simulink model "testEmplanner_cs -copy"  (R2021b)
settings: Solver=ode5  StartTime=0.0  StopTime=30  FixedStep=1/1000  RelTol=1e-3
PreLoadFcn:
  | mbxruntime.callbacks.PreLoadFcn(bdroot);
PostLoadFcn:
  | mbxruntime.callbacks.PostLoadFcn(bdroot);
InitFcn:
  | mbxruntime.callbacks.InitFcn(bdroot);
StartFcn:
  | mbxruntime.callbacks.StartFcn(bdroot);
StopFcn:
  | mbxruntime.callbacks.StopFcn(bdroot);
model workspace (MAT data in the model file):
  mbox_table : object (value not decoded)
  model_closed = 0
  sim_status = 0
values from neighbouring files (symbols this model uses):
  c_factor = 43.75    [emplanner_init.m]
  cf = -175016    [emplanner_init.m]
  cr = -130634    [emplanner_init.m]
  global_path_x = [-1.1448 -0.145417744933 0.852705365581 1.84955224935 2.84511712279 3.83939835808 4.83239585569 5.82411007764 6.81454169183 7.80369144113 8.79156009523 9.77814843293 ... (3001 elements, 3001x1)]    [global_path.mat]
  global_path_y = [14.6488 14.6488 14.6488 14.6488 14.6488 14.6488 14.6488 14.6488 14.6488 14.6488 14.6488 14.6488 ... (3001 elements, 3001x1)]    [global_path.mat]
  KD_PID_distance = 0.0    (= 0)    [emplanner_init.m]
  KD_PID_speed = 0    [emplanner_init.m]
  KI_PID_distance = 0.0    (= 0)    [emplanner_init.m]
  KI_PID_speed = 0    [emplanner_init.m]
  KP_PID_distance = 0.5    [emplanner_init.m]
  KP_PID_speed = 1.8    [emplanner_init.m]
  la = 1.265    [emplanner_init.m]
  lb = 2.947-1.265    (= 1.682)    [emplanner_init.m]
  LQR_K1 = k(:,1)'    [emplanner_init.m]
  LQR_K2 = k(:,2)'    [emplanner_init.m]
  LQR_K3 = k(:,3)'    [emplanner_init.m]
  LQR_K4 = k(:,4)'    [emplanner_init.m]
  m = 2020    [emplanner_init.m]
  rack_displacement = [-39.14 , -37.2 , -35.29 , -33.43 , -31.6 , -29.81 , -28.06 , -26.34 , -24.66 ,      -23.01 , -21.38 , -19.79 , -18.23 , -16.69 , -15.18 , -13.7 , -12.23 , -10.8 , -9.38 , -7.98 ,     -6.61 , -5.25 , -3.91 , -2.59 , -1.29 , 0 , 1.27 , 2.54 , 3.78 , 5.02 , 6.24 , 7.46 , 8.66 ,      9.86 , 11.05 , 12.24 , 13.41 , 14.59 , 15.76 , 16.92 , 18.09 , 19.25 , 20.42 , 21.59 , 22.76 ,      23.93 , 25.11 , 26 ...(+26 chars)    [emplanner_init.m]
  right_wheel_ground = [-70 ,-67.2 , -64.4 , -61.6 , -58.8 , -56 , -53.2 , -50.4 , -47.6 , -44.8 , -42 ,      -39.2 , -36.4 , -33.6 , -30.8 , -28 , -25.2 , -22.4 , -19.6 , -16.8 , -14 , -11.2 , -8.4 , -5.6 ,      -2.8 , 0 , 2.8 , 5.6 , 8.4 , 11.2 , 14 , 16.8 , 19.6 , 22.4 , 25.2 , 28 , 30.8 , 33.6 , 36.4 ,      39.2 , 42 , 44.8 , 47.6 , 50.4 , 53.2 , 56 , 58.8 , 61.6 , 64.4 , 67.2 , 70 ]    [emplanner_init.m]
  vx_break_point = zeros(1,5000)    [emplanner_init.m]
undefined symbols (not defined in the file or in its folder): aubr, DiscIntNeverNeededParam, tablebr, vubr, warningInitialVelocity, x0
libraries: simulink x19, PreScanSimulinkLibrary x11, simulink_extras x6, Solver_SF x1
(part 8 of 8)

== matlab function testEmplanner_cs -copy/Audi_A8_Sedan_1/decision&planning module/EM Planner/MATLAB Function ==
  data: obs_s_set input; dp_path_s output; obs_l_set input; plan_start_s input; plan_start_l input; plan_start_dl input; plan_start_ddl input; w_cost_collision input; w_cost_smooth_dl input; w_cost_smooth_ddl input; w_cost_smooth_dddl input; w_cost_ref input; row input; col input; sample_s input; sample_l input; dp_path_l output
function [dp_path_s,dp_path_l] = fcn(obs_s_set,obs_l_set,plan_start_s,plan_start_l,plan_start_dl,...
	plan_start_ddl,w_cost_collision,w_cost_smooth_dl,w_cost_smooth_ddl,w_cost_smooth_dddl,w_cost_ref,row,col,sample_s,sample_l)
% 该函数为路径决策算法动态规划的主函数
% 输入：obs s l set 筛选后的障碍物的sl信息
% 		plan_start s l dl ddl 规划起点的信息
% 		w_cost_obs,w_cost_smooth_dl,w_cost_smooth_ddl,w_cost_smooth_dddl,w_cost_ref 动态规划代价权重
% 		row col 动态规划采样点的行数和列数
% 		sample_s,sample_l 采样点s l长度
%输出：dp_path_l，dp_path_s 动态规划的路径s l

%动态规划最优的数据结构是结构体矩阵，但是simulink不支持结构体矩阵，所以动态规划算法写的相对难理解

%声明二维矩阵变量node_cost, node_cost(i,j)表示从起点出发,到i行，j列节点的最小代价为node_cost(i,j)
node_cost = ones(row,col) * inf;%初始化为无穷大
%声明二维矩阵变量 pre_node_index pre_node_index(i,j)表示从起点到行j列的节点的最优路径中前一个节点的行号为
%pre_node_index(i,j)
%例如：比如一条最优的路径为 起点--> node(1,1) --> node(2,2) --> node(3,3)
%则pre_node_index(3,3) = 2 （最优路径的前一个节点是node(2,2),取的是他的行号，列号是直接减1即可）
%  pre_node_index(2,2) = 1 (最优路径的前一个节点node(1,1)取它的行号，列号直接减去1即可)
%  pre_node_index(1,1) = 0 (起点的行号默认是0)

% 其实pre_node_index就是当我找到最小代价的路径后，从终点到起点反向选择出的最优路径
% 如果用结构体矩阵完全没有必要弄得这么麻烦，但是simulink不支持

pre_node_index = zeros(row,col);%初始化，所有节点上的最优节点的行号都是0，也就是起点

%先计算从起点到第一列的cost

for i = 1: row
	node_cost(i,1) = CalcStartCost(plan_start_s,plan_start_l,plan_start_dl,...
		plan_start_ddl,i,sample_s,sample_l,w_cost_collision,w_cost_smooth_dl,...
		w_cost_smooth_ddl,w_cost_smooth_dddl,w_cost_ref,obs_s_set,obs_l_set,row);
end
% 动态规划的主函数，从第二列开始
% 计算列，然后计算行
for j = 2 : col 
	for i = 1 : row
		% 计算当前的node(i,j) 的s,l
		cur_node_s = plan_start_s + j * sample_s;
		cur_node_l = ((row + 1) / 2 - i) * sample_l;
		% 遍历前一列的节点
		for k = 1 : row 
			% 计算前一列节点的 s l 
			pre_node_s = plan_start_s + (j - 1) * sample_s;
			pre_node_l = ((row + 1) / 2  - k) * sample_l;
			cost_neighbour = CalcNeighbourCost(pre_node_s,pre_node_l,cur_node_s,cur_node_l,w_cost_collision,...
				w_cost_smooth_dl,w_cost_smooth_ddl,w_cost_smooth_dddl,w_cost_ref,obs_s_set,obs_l_set);
			pre_min_cost = node_cost(k,j-1);
			%起点到node_cost(i,j)的最小代价 为node_cost(k,j-1)
			%再加上 node(k,j-1)到node(i,j)的代价 (k = 1,2,3,4 ... row)中最小的
			cost_temp = pre_min_cost + cost_neighbour;
			if cost_temp < node_cost(i,j)
				node_cost(i,j) = cost_temp;
				%把最优的路径上一列的行号记录下来
				pre_node_index(i,j) = k;
			end
		end
	end
end
% 找到node_cost最后一列中，cost最小的，记代价最小的行号为index
index = 0;
min_cost = inf;
for i = 1 :row
	if node_cost(i,end) < min_cost
		min_cost = node_cost(i,end);
		index = i;
	end
end	

%动态规划的最优路径初始化
dp_node_list_row = zeros(col,1);
% 从后往前逆推
cur_index = index;
for i = 1 : col
	%记录cur_index 前面节点的行号
	pre_index = pre_node_index(cur_index,col - i + 1);
	%把cur_index放到dp_node_list的对应位置
	dp_node_list_row(col - i + 1) = cur_index;
	% 再把pre_index 赋给cur_index 进行下一步递推
	cur_index = pre_index;
end

%输出初始化，由于事先不知道横纵向的采样列数，因此需要做缓冲
dp_path_s = ones(15,1) * -1;
dp_path_l = ones(15,1) * -1;
for i = 1 : col 
	dp_path_s(i) = plan_start_s + i * sample_s;
	dp_path_l(i) = ((row + 1) / 2 - dp_node_list_row(i)) * sample_l;
end
end


function cost = CalcNeighbourCost(pre_node_s,pre_node_l,cur_node_s,cur_node_l,w_cost_collision,...
				w_cost_smooth_dl,w_cost_smooth_ddl,w_cost_smooth_dddl,w_cost_ref,obs_s_set,obs_l_set)
% 该函数将计算相邻两个节点之间的cost
	start_l = pre_node_l;
	start_dl = 0;
	start_ddl = 0;
    end_l = cur_node_l;
	end_dl = 0;
	end_ddl = 0;
	start_s = pre_node_s;
	end_s = cur_node_s;
	coeff = CalcQuinticCoeffient(start_l,start_dl,start_ddl,end_l,end_dl,end_ddl,start_s,end_s);
	a0 = coeff(1);
	a1 = coeff(2);
	a2 = coeff(3);
	a3 = coeff(4);
	a4 = coeff(5);
	a5 = coeff(6);
	% 取10个点计算cost
	ds = zeros(10,1);
	l = zeros(10,1);
	dl = zeros(10,1);
	ddl = zeros(10,1);
	dddl = zeros(10,1);
	for i = 1 : 10
		ds(i) = start_s + (i - 1) * (end_s - start_s) / 10;
	end

	l = a0 * ones(10,1) + a1 * ds + a2 * ds.^2 + a3 * ds.^3 + a4 * ds.^4 + a5  * ds.^5;
	dl = a1 * ones(10,1) + 2 * a2 * ds + 3 * a3 * ds.^2 + 4 * a4 * ds.^3 + 5 * ds.^4;
	ddl = 2 * a2 * ones(10,1) + 6 * a3 * ds + 12 * a4 * ds.^2 + 20 * a5 * ds.^3;
	dddl = 6 * a3 * ones(10,1) + 24 * a4 * ds + 60 * a5 * ds.^2 ;
	cost_smooth = w_cost_smooth_dl * (dl' * dl) + w_cost_smooth_ddl * (ddl' * ddl) + w_cost_smooth_dddl * (dddl' * dddl);
	for i = 1 : length(ddl)
		if abs(ddl(i) > 0.5 || abs(atan(dl(i)))) > 0.4 * pi
			cost_smooth = cost_smooth + 1e7;
			break;
		end
	end
	% 参考线代价，为离参考线的距离的代价
	cost_ref = w_cost_ref * (l' * l);

	% 障碍物代价 首先设置为0 ,简化近似，只认为障碍物是一个点
	cost_collision = 0;
	for i = 1 : length(obs_s_set)
		if isnan(obs_s_set(i))
			break;
		end
		dlon = ones(10,1) * obs_s_set(i) - ds;
		dlat = ones(10,1) * obs_l_set(i) - l;
		% 这里做了非常简化的质点模型，认为障碍物就是一点，动态规划就是为了开辟一个凸空间，没必要考虑这么细致，
		% 可以在二次规划中（速度规划）进行细化
		square_d = dlon.^2 + dlat.^2; % 近似处理，真正是欧式空间里的距离和
		%一个障碍物的碰撞代价，如果多个障碍物就是多个障碍物代价叠加
		cost_collision_once = CalcObsCost(w_cost_collision,square_d); 
		cost_collision = cost_collision + cost_collision_once;

		% 判断障碍物的左右
		v1 = [ds(end);l(end)] - [ds(1);l(1)];
		v2 = [obs_s_set(i);obs_l_set(i)] - [ds(1);l(1)];
		flag = v1(1)*v2(2) - v1(2)*v2(1);
		if flag < 0 && cost_collision > 0 
			cost_collision = cost_collision - 1000;
		end
	end
	% 总代价 =  碰撞代价 + 平滑代价 + 参考线代价
	cost = cost_collision + cost_smooth + cost_ref;
end

function cost = CalcStartCost(begin_s,begin_l,begin_dl,begin_ddl,cur_node_row,sample_s,sample_l,w_cost_collision,...
	w_cost_smooth_dl,w_cost_smooth_ddl,w_cost_smooth_dddl,w_cost_ref,obs_s_set,obs_l_set,row)
	%该函数将计算起点到第一层的cost
	start_l = begin_l;
	start_dl = begin_dl;
	start_ddl = begin_ddl;
	% . . .
	% . . . row = 3 中间的行号 = (row + 1) / 2 = 2
 	% . . .
    end_l = ((row + 1) / 2 - cur_node_row) * sample_l;
	end_dl = 0;
	end_ddl = 0;
	start_s = begin_s;
	end_s = begin_s + sample_s;
	coeff = CalcQuinticCoeffient(start_l,start_dl,start_ddl,end_l,end_dl,end_ddl,start_s,end_s);
	a0 = coeff(1);
	a1 = coeff(2);
	a2 = coeff(3);
	a3 = coeff(4);
	a4 = coeff(5);
	a5 = coeff(6);
	% 取10个点计算cost
	ds = zeros(10,1);
	l = zeros(10,1);
	dl = zeros(10,1);
	ddl = zeros(10,1);
	dddl = zeros(10,1);
	for i = 1 : 10
		ds(i) = start_s + (i - 1) * sample_s / 10;
	end

	l = a0 * ones(10,1) + a1 * ds + a2 * ds.^2 + a3 * ds.^3 + a4 * ds.^4 + a5  * ds.^5;
	dl = a1 * ones(10,1) + 2 * a2 * ds + 3 * a3 * ds.^2 + 4 * a4 * ds.^3 + 5 * ds.^4;
	ddl = 2 * a2 * ones(10,1) + 6 * a3 * ds + 12 * a4 * ds.^2 + 20 * a5 * ds.^3;
	dddl = 6 * a3 * ones(10,1) + 24 * a4 * ds + 60 * a5 * ds.^2 ;
	cost_smooth = w_cost_smooth_dl * (dl' * dl) + w_cost_smooth_ddl * (ddl' * ddl) + w_cost_smooth_dddl * (dddl' * dddl);
	for i = 1 : length(ddl)
		if abs(ddl(i) > 0.5 || abs(atan(dl(i)))) > 0.4 * pi
			cost_smooth = cost_smooth + 1e7;
			break;
		end
	end
	% 参考线代价，为离参考线的距离的代价
	cost_ref = w_cost_ref * (l' * l);

	% 障碍物代价 首先设置为0 ,简化近似，只认为障碍物是一个点
	cost_collision = 0;
	for i = 1 : length(obs_s_set)
		if isnan(obs_s_set(i))
			break;
		end
		dlon = ones(10,1) * obs_s_set(i) - ds;
		dlat = ones(10,1) * obs_l_set(i) - l;
		% 这里做了非常简化的质点模型，认为障碍物就是一点，动态规划就是为了开辟一个凸空间，没必要考虑这么细致，
		% 可以在二次规划中（速度规划）进行细化
		square_d = dlon.^2 + dlat.^2; % 近似处理，真正是欧式空间里的距离和
		%一个障碍物的碰撞代价，如果多个障碍物就是多个障碍物代价叠加
		cost_collision_once = CalcObsCost(w_cost_collision,square_d); 
		cost_collision = cost_collision + cost_collision_once;
		% 判断障碍物的左右
        v1 = [ds(end);l(end)] - [ds(1);l(1)];
        v2 = [obs_s_set(i);obs_l_set(i)] - [ds(1);l(1)];
        flag = v1(1)*v2(2) - v1(2)*v2(1);
        if flag < 0 && cost_collision > 0
            cost_collision = cost_collision - 1000;
        end
	end

	% 总代价 =  碰撞代价 + 平滑代价 + 参考线代价
	cost = cost_collision + cost_smooth + cost_ref;
end

function obs_cost = CalcObsCost(w_cost_collision,square_d)
	% 该函数将计算障碍物的距离代价
	% 暂时定义：超过4米的cost为0 在4到3米的cost 为 1000 / square_d,在小于3米的cost为 w_cost_collision
	%cost = 0;
	%for i = 1 : length(square_d)
	%	if (square_d(i) < 16 && square_d(i) >9)
	%		cost = cost + 500 / square_d(i);
	%	elseif(square_d(i) <= 9)
	%		cost = cost + w_cost_collision;
	%	end
	%end
	min_d = inf;
	for i = 1 : length(square_d)
		min_d = min(min_d,square_d(i));
	end

	obs_cost = w_cost_collision * 10 ^ (-min_d/3);
end


function coeff = CalcQuinticCoeffient(start_l,start_dl,start_ddl,end_l,end_dl,end_ddl,start_s,end_s)
	% l = a0 + a1 * s + a2 * s^2 + a3 * s^3 + a4 * s^4 + a5 * s^5;
	% l' = a1 + 2 * a2 * s + 3 * a3 * s^2 + 4 * a4 * s^3 + 5 * a5 * s^4;
	% l'' = 2 * a2 + 6 * a3 * s + 12 * a4 * s^2 + 20 * a5 * s^3;
	start_s2 = start_s * start_s;
	start_s3 = start_s2 * start_s;
	start_s4 = start_s3 * start_s;
	start_s5 = start_s4 * start_s;

	end_s2 = end_s * end_s;
	end_s3 = end_s2 * end_s;
	end_s4 = end_s3 * end_s;
	end_s5 = end_s4 * end_s;
	% 构造A B矩阵，然后求方程的系数即可

	A = [ 1, start_s, start_s2,  start_s3,   start_s4,   start_s5;
		  0 , 1     , 2*start_s, 3*start_s2, 4*start_s3,  5*start_s4;
		  0 , 0     , 2        , 6*start_s,  12*start_s2, 20*start_s3;
		  1, end_s, end_s2,  end_s3,   end_s4,   end_s5;
		  0 , 1     , 2*end_s, 3*end_s2, 4*end_s3,  5*end_s4;
		  0 , 0     , 2         , 6*end_s,  12*end_s2, 20*end_s3;
		];
	B = [ start_l;
		  start_dl;
		  start_ddl;
		  end_l;
		  end_dl;
		  end_ddl;
		];
	coeff = A \ B;
end

== matlab function testEmplanner_cs -copy/Audi_A8_Sedan_1/decision&planning module/EM Planner/MATLAB Function1 ==
  data: dp_path_s_init input; dp_path_s_final output; dp_path_l_init input; plan_start_s input; plan_start_l input; plan_start_dl input; plan_start_ddl input; dp_path_l_final output; dp_path_dl_final output; dp_path_ddl_final output
function [dp_path_s_final,dp_path_l_final,dp_path_dl_final,dp_path_ddl_final] = ... 
	fcn(dp_path_s_init,dp_path_l_init,plan_start_s,plan_start_l,plan_start_dl,plan_start_ddl)
% 该函数将增密dp_path_s,dp_path_l
% 由于事先不知道动态规划采样的行和列，也就不知道动态规划计算的曲线有多长，因此需要做缓冲
% 每1“米” 采样一个点，一共60个
ds = 1;
% 输出初始化
dp_path_s_final = ones(60,1) * nan;
dp_path_l_final = ones(60,1) * nan;
dp_path_dl_final = ones(60,1) * nan;
dp_path_ddl_final = ones(60,1) * nan;

% 设置五次多项式的起点
start_s = plan_start_s;
start_l = plan_start_l;
start_dl = plan_start_dl;
start_ddl = plan_start_ddl;

s_cur = [];
l_temp = [];
dl_temp = [];
ddl_temp = [];

for i = 1 : length(dp_path_s_init)
	if dp_path_s_init == -1 
		break;
	end
	for j = 1 : 1000
		% 采样s
		s_node = start_s + ds * (j - 1);
		if s_node < dp_path_s_init(i)
			s_cur = [s_cur,s_node];% 矩阵动态扩容
		else
			break;
		end

	end
	end_s = dp_path_s_init(i);
	end_l = dp_path_l_init(i);
	end_dl = 0;
	end_ddl = 0;
	coeff = CalcQuinticCoeffient(start_l,start_dl,start_ddl,end_l,end_dl,end_ddl,start_s,end_s);
	a0 = coeff(1);
	a1 = coeff(2);
	a2 = coeff(3);
	a3 = coeff(4);
	a4 = coeff(5);
	a5 = coeff(6);
	l = a0 * ones(1,length(s_cur)) + a1 * s_cur + a2 * s_cur.^2 + a3 * s_cur.^3 +...
		a4 * s_cur.^4 + a5 * s_cur.^5 ;
	dl = a1 * ones(1,length(s_cur)) + 2 * a2 * s_cur + 3 * a3 * s_cur.^2 + ...
		4 * a4 * s_cur.^3 + 5 * a5 * s_cur.^4;
	ddl = 2 * a2 * ones(1,length(s_cur)) + 6 * a3 * s_cur + ...
		12 * a4 * s_cur.^2 + 20 * a5 * s_cur.^3;
	% 把 l dl ddl 的结果保存
	l_temp = [l_temp,l];
	dl_temp = [dl_temp,dl];
	ddl_temp = [ddl_temp,ddl];
	% end的值 赋值给start做下一步循环使用
	start_s = end_s;
	start_l = end_l;
	start_dl = end_dl;
	start_ddl = end_ddl;
	s_cur = [];% 清空临时数组
end

	for k = 1 : length(l_temp)
		if k == 61 
			break;
		end

		dp_path_s_final(k) = plan_start_s + ds * (k - 1);
		dp_path_l_final(k) = l_temp(k);
		dp_path_dl_final(k) = dl_temp(k);
		dp_path_ddl_final(k) = ddl_temp(k);

	end

end


function coeff = CalcQuinticCoeffient(start_l,start_dl,start_ddl,end_l,end_dl,end_ddl,start_s,end_s)
	% l = a0 + a1 * s + a2 * s^2 + a3 * s^3 + a4 * s^4 + a5 * s^5;
	% l' = a1 + 2 * a2 * s + 3 * a3 * s^2 + 4 * a4 * s^3 + 5 * a5 * s^4;
	% l'' = 2 * a2 + 6 * a3 * s + 12 * a4 * s^2 + 20 * a5 * s^3;
	start_s2 = start_s * start_s;
	start_s3 = start_s2 * start_s;
	start_s4 = start_s3 * start_s;
	start_s5 = start_s4 * start_s;

	end_s2 = end_s * end_s;
	end_s3 = end_s2 * end_s;
	end_s4 = end_s3 * end_s;
	end_s5 = end_s4 * end_s;
	% 构造A B矩阵，然后求方程的系数即可

	A = [ 1, start_s, start_s2,  start_s3,   start_s4,   start_s5;
		  0 , 1     , 2*start_s, 3*start_s2, 4*start_s3,  5*start_s4;
		  0 , 0     , 2        , 6*start_s,  12*start_s2, 20*start_s3;
		  1, end_s, end_s2,  end_s3,   end_s4,   end_s5;
		  0 , 1     , 2*end_s, 3*end_s2, 4*end_s3,  5*end_s4;
		  0 , 0     , 2       , 6*end_s,  12*end_s2, 20*end_s3;
		];
	B = [ start_l;
		  start_dl;
		  start_ddl;
		  end_l;
		  end_dl;
		  end_ddl;
		];
	coeff = A \ B;
end

== matlab function testEmplanner_cs -copy/Audi_A8_Sedan_1/decision&planning module/EM Planner/MATLAB Function2 ==
  data: s_set input; x_set output; l_set input; dl_set input; ddl_set input; frenet_path_x input; frenet_path_y input; frenet_path_heading input; frenet_path_kappa input; index2s input; y_set output; heading_set output; kappa_set output
function [x_set,y_set,heading_set,kappa_set] = ...
	fcn(s_set,l_set,dl_set,ddl_set,frenet_path_x,frenet_path_y,frenet_path_heading,frenet_path_kappa,index2s)
% 通用算法 frenet 转Cartesian
% 由于不知道有多少个(s,l)要转化成直角坐标，因此需要做缓冲
% 输出初始化
 	x_set = ones(600,1) * nan;
 	y_set = ones(600,1) * nan;
 	heading_set = ones(600,1) * nan;
 	kappa_set = ones(600,1) * nan;
 	for i = 1 : length(s_set)
 		if isnan(s_set(i))
 			break;
 		end
 		% 计算（s,l) 在frenet坐标轴上的投影
 		[proj_x,proj_y,proj_heading,proj_kappa] = CalcProjPoint(s_set(i),frenet_path_x,frenet_path_y,frenet_path_heading,...
			frenet_path_kappa,index2s);
		nor = [-sin(proj_heading); cos(proj_heading)];
		point = [proj_x;proj_y] + l_set(i) * nor;
		x_set(i) = point(1);
		y_set(i) = point(2);
		heading_set(i) = proj_heading + atan(dl_set(i) / (1 - proj_kappa * l_set(i)));
		% 近似认为 kappa’ == 0；frenet 转cartesian公式，见csdn的公式
		kappa_set(i) = ((ddl_set(i) + proj_kappa * dl_set(i) * tan(heading_set(i) - proj_heading)) *...
			(cos(heading_set(i) - proj_heading)^2) / (1 - proj_kappa * l_set(i)) + proj_kappa) *...
			cos(heading_set(i) - proj_heading) / (1 - proj_kappa * l_set(i));
 	end

end

% path 从自然坐标系转到直角坐标系，才能发给控制去使用
% 最重要是要找投影点


function[proj_x,proj_y,proj_heading,proj_kappa] = CalcProjPoint(s,frenet_path_x,frenet_path_y,frenet_path_heading,...
	frenet_path_kappa,index2s)
% 该函数啊将计算在frenet坐标系下，点(s,l) 在frenet坐标轴的投影的直角坐标(proj_x,proj_y,proj_heading,proj_kappa)
% 先找到匹配点的编号
	match_index = 1;
	while index2s(match_index) < s
		match_index = match_index + 1;
	end
	match_point = [frenet_path_x(match_index);frenet_path_y(match_index)];
	match_point_heading = frenet_path_heading(match_index);
	match_point_kappa = frenet_path_kappa(match_index);
	ds = s - index2s(match_index);
	
	% 根据匹配点计算投影点算法
	match_tor = [cos(match_point_heading);sin(match_point_heading)];
	proj_point = match_point + ds * match_tor;
	proj_heading = match_point_heading + ds * match_point_kappa;
	proj_kappa = match_point_kappa;
	proj_x = proj_point(1);
	proj_y = proj_point(2);
end

== matlab function testEmplanner_cs -copy/Audi_A8_Sedan_1/decision&planning module/EM Planner/calc path length and map between point and s ==
  data: trajectory_x input; path_s_end output; trajectory_y input; path_s output
function [path_s_end,path_s] = fcn(trajectory_x,trajectory_y)
% 该函数将计算以trajectory的s 与 x y 的对应关系，可以看作是trajectory index2s
n = length(trajectory_x);
path_s = zeros(n,1);
sum = 0;
for i = 2:length(trajectory_x)
    if isnan(trajectory_x(i))
        break;
    end
    sum = sum + sqrt((trajectory_x(i) - trajectory_x(i-1))^2 + (trajectory_y(i) - trajectory_y(i-1))^2);
    path_s(i) = sum;
end
% 计算出trajectory的长度
if i == n
    path_s_end = path_s(end);
else
    % 因为循环的退出条件为isnan(trajectory_x(i)) 所以 i 所对应的数为 nan 
    path_s_end = path_s(i - 1);
end

== matlab function testEmplanner_cs -copy/Audi_A8_Sedan_1/decision&planning module/EM Planner/increase st point count ==
  data: s_init input; s output; s_dot_init input; s_dot2_init input; relative_time_init input; s_dot output; s_dot2 output; relative_time output
function [s,s_dot,s_dot2,relative_time] = fcn(s_init,s_dot_init,s_dot2_init,relative_time_init)
%该函数将增密s s_dot s_dot2
% 为什么需要增密，因为控制的执行频率是规划的10倍，轨迹点如果不够密，必然会导致规划效果不好
% 但是若在速度二次规划中点取的太多，会导致二次规划的矩阵规模太大计算太慢
% 所以方法是在二次规划中选取少量的点优化完毕后，在用此函数增密
T = relative_time_init(end);
n = 401;
dt = T/(n-1);
s = zeros(n,1);
s_dot = zeros(n,1);
s_dot2 = zeros(n,1);
relative_time = zeros(n,1);
for i = 1:n
    current_t = (i-1)*dt;
    for j = 1:length(relative_time_init)-1
        if relative_time_init(j) <= current_t && relative_time_init(j+1) > current_t
            break;
        end
    end
    x = current_t - relative_time_init(j);
    s(i) = s_init(j) + s_dot_init(j)*x + (1/3)*s_dot2_init(j)*x^2 + (1/6)*s_dot2_init(j+1)*x^2; 
    s_dot(i) = s_dot_init(j) + 0.5*s_dot2_init(j)*x + 0.5*s_dot2_init(j+1)*x;
    s_dot2(i) = s_dot2_init(j) + (s_dot2_init(j+1) - s_dot2_init(j))*x/(relative_time_init(j+1) - relative_time_init(j));
    relative_time(i) = current_t;
end

== matlab function testEmplanner_cs -copy/Audi_A8_Sedan_1/decision&planning module/EM Planner/path and speed merge ==
  data: s input; trajectory_x output; s_dot input; s_dot2 input; relative_time input; current_time input; path_s input; trajectory_x_init input; trajectory_y_init input; trajectory_heading_init input; trajectory_kappa_init input; trajectory_y output; trajectory_heading output; trajectory_kappa output; trajectory_speed output; trajectory_accel output; trajectory_time output
function [trajectory_x,trajectory_y,trajectory_heading,trajectory_kappa,trajectory_speed,trajectory_accel,trajectory_time] = ...
    fcn(s,s_dot,s_dot2,relative_time,current_time,path_s,trajectory_x_init,trajectory_y_init,trajectory_heading_init,trajectory_kappa_init)
% 该函数将合并path和speed
% 由于path 是 60个点，speed 有 401个点，合并后，path和speed有401个点，因此需要做插值
n = 401;
trajectory_x = zeros(n,1);
trajectory_y = zeros(n,1);
trajectory_heading = zeros(n,1);
trajectory_kappa = zeros(n,1);
trajectory_speed = zeros(n,1);

trajectory_accel = zeros(n,1);
index = 1;
% 由于trajectory_x_init中不是所有的值都有效，(有nan) 所以要找到有效值的范围
while ~isnan(trajectory_x_init(index)) 
    index = index + 1;
end
index = index - 1;
trajectory_time = zeros(n,1);
for i = 1:n-1
    %interp1 线性插值
    % 若 x = [1,2] y = [3,4]
    %interp1(x,y,1.5) 会得到3.5
    %interp1 的缺点是 在端点或超过端点的，结果为nan
    % interp1(x,y,2) 不会等于4 而是会等于nan
    % interp1(x,y,6) 也会等于nan，所以在端点处要单独处理
    trajectory_x(i) = interp1(path_s(1:index),trajectory_x_init(1:index),s(i));
    trajectory_y(i) = interp1(path_s(1:index),trajectory_y_init(1:index),s(i));
    trajectory_heading(i) = interp1(path_s(1:index),trajectory_heading_init(1:index),s(i));
    trajectory_kappa(i) = interp1(path_s(1:index),trajectory_kappa_init(1:index),s(i));
    trajectory_time(i) = relative_time(i) + current_time;%速度规划会得到相对时间，转换成绝对时间
    trajectory_speed(i) = s_dot(i);
    trajectory_accel(i) = s_dot2(i);
end
% 端点单独处理
trajectory_x(end) = trajectory_x_init(end);
trajectory_y(end) = trajectory_y_init(end);
trajectory_heading(end) = trajectory_heading_init(end);
trajectory_kappa(end) = trajectory_kappa_init(end);
trajectory_time(end) = relative_time(end) + current_time;
trajectory_speed(end) = s_dot(end);
trajectory_accel(end) = s_dot2(end);

== matlab function testEmplanner_cs -copy/Audi_A8_Sedan_1/decision&planning module/EM Planner/stitch trajectory ==
  data: trajectory_x input; trajectory_x_final output; trajectory_y input; trajectory_heading input; trajectory_kappa input; trajectory_speed input; trajectory_accel input; trajectory_time input; stitch_x input; stitch_y input; stitch_heading input; stitch_kappa input; stitch_speed input; stitch_accel input; stitch_time input; trajectory_y_final output; trajectory_heading_final output; trajectory_kappa_final output; trajectory_speed_final output; trajectory_accel_final output; trajectory_time_final output
function [trajectory_x_final,trajectory_y_final,trajectory_heading_final,trajectory_kappa_final,...
          trajectory_speed_final,trajectory_accel_final,trajectory_time_final] = fcn(trajectory_x,...
          trajectory_y,trajectory_heading,trajectory_kappa,trajectory_speed,trajectory_accel,trajectory_time,...
          stitch_x,stitch_y,stitch_heading,stitch_kappa,stitch_speed,stitch_accel,stitch_time)
% 轨迹拼接，把stitch trajectory 拼到规划完成的轨迹上
n = 401 + 20;
trajectory_x_final = zeros(n,1);
trajectory_y_final = zeros(n,1);
trajectory_heading_final = zeros(n,1);
trajectory_kappa_final = zeros(n,1);
trajectory_speed_final = zeros(n,1);
trajectory_accel_final = zeros(n,1);
trajectory_time_final = zeros(n,1);

trajectory_x_final = [stitch_x;trajectory_x];
trajectory_y_final = [stitch_y;trajectory_y];
trajectory_heading_final = [stitch_heading;trajectory_heading];
trajectory_kappa_final = [stitch_kappa;trajectory_kappa];
trajectory_speed_final = [stitch_speed;trajectory_speed];
trajectory_accel_final = [stitch_accel;trajectory_accel];
trajectory_time_final = [stitch_time;trajectory_time];

== matlab function testEmplanner_cs -copy/Audi_A8_Sedan_1/control module/MATLAB Function ==
  data: trajectory_x input; xr output; trajectory_y input; trajectory_heading input; trajectory_kappa input; trajectory_speed input; trajectory_accel input; trajectory_time input; current_time input; yr output; thetar output; kappa output; vr output; ar output
function [xr,yr,thetar,kappa,vr,ar] = fcn(trajectory_x,trajectory_y,trajectory_heading,...
	trajectory_kappa,trajectory_speed,trajectory_accel,trajectory_time,current_time)
% 该函数根据规划的轨迹计算出期望跟踪的点
% 由于控制也是有延迟的，所以控制发出的期望跟踪点是current_time + 0.01;
control_time = current_time + 0.01;
% 规划发出的轨迹有一部分是拼接的，在刚启动的时候，stitch_time = -1,因此要它先去掉
start_index = 1;
while (trajectory_time(start_index) == -1)
	start_index = start_index + 1;
end	
% 使用interp1插值计算得到xr yr thethar kappa vr ar 要在两个边界中间，不能包括端点
% 由于interp1在端点会得到nan，因此要防一手
% 解释，为什么trajectory_time(start_index) ~= 0
% 因为在刚开始启动时规划先执行（100ms）,当规划完毕的时候，控制已经执行了10次
% 那么在最开始的时候，规划还给控制发送结果，控制已经执行了10次，在这10次中，控制跟踪的轨迹是空轨迹
% simulink 空轨迹是 0，0，0，0 ... ,这样trajectory_time，也全是0，trajectory_time 不单调递增
% 而interp1(x,y,x0)，要求x是单调递增，否则会报错

if control_time > trajectory_time(start_index) && trajectory_time(start_index) ~= 0
	xr = interp1(trajectory_time(start_index:end),trajectory_x(start_index:end),control_time);
	yr = interp1(trajectory_time(start_index:end),trajectory_y(start_index:end),control_time);	
	thetar = interp1(trajectory_time(start_index:end),trajectory_heading(start_index:end),control_time);	
	kappa = interp1(trajectory_time(start_index:end),trajectory_kappa(start_index:end),control_time);	
	vr = interp1(trajectory_time(start_index:end),trajectory_speed(start_index:end),control_time);
	ar = interp1(trajectory_time(start_index:end),trajectory_accel(start_index:end),control_time);				
else
	xr = trajectory_x(start_index);
	yr = trajectory_y(start_index);	
	thetar = trajectory_heading(start_index);	
	kappa = trajectory_kappa(start_index);	
	vr = trajectory_speed(start_index);
	ar = trajectory_accel(start_index);	
end

== matlab function testEmplanner_cs -copy/Audi_A8_Sedan_1/decision&planning module/EM Planner/plot ==
  data: dp_s input; dp_l input; qp_l input; l_min input; l_max input; obs_s_set input; obs_l_set input; start_s input; start_l input; start_dl input
function  fcn(dp_s,dp_l,qp_l,l_min,l_max,obs_s_set,obs_l_set,start_s,start_l,start_dl)
coder.extrinsic("plot","axis","figure","drawnow","cla","fill");

obs_length = 5;
obs_width = 2;
host_l = 6;
host_w = 1.63;
cla;
host_p1_l = start_l + sin(atan(start_dl)) * host_l /2 + host_w/2 * cos(atan(start_dl));
host_p1_s = start_s + cos(atan(start_dl)) * host_l /2 - host_w/2 * sin(atan(start_dl));
host_p2_l = start_l + sin(atan(start_dl)) * host_l /2 - host_w/2 * cos(atan(start_dl));
host_p2_s = start_s + cos(atan(start_dl)) * host_l /2 + host_w/2 * sin(atan(start_dl));
host_p3_l = start_l - sin(atan(start_dl)) * host_l /2 + host_w/2 * cos(atan(start_dl));
host_p3_s = start_s - cos(atan(start_dl)) * host_l /2 - host_w/2 * sin(atan(start_dl));
host_p4_l = start_l - sin(atan(start_dl)) * host_l /2 - host_w/2 * cos(atan(start_dl));
host_p4_s = start_s - cos(atan(start_dl)) * host_l /2 + host_w/2 * sin(atan(start_dl));
host_area_x = [host_p1_s;host_p2_s;host_p4_s;host_p3_s];
host_area_y = [host_p1_l;host_p2_l;host_p4_l;host_p3_l];
fill(host_area_x,host_area_y,[0 1 1]);
hold on
plot(dp_s,dp_l,'r');

plot(dp_s,qp_l,'b');
plot(dp_s,l_min,dp_s,l_max);
axis([-8 70 -10 10]);

for i = 1:length(obs_s_set)
    if isnan(obs_s_set(i))
        break;
    end
    obs_p1_s = obs_s_set(i) + obs_length/2;
    obs_p1_l = obs_l_set(i) + obs_width/2;
    obs_p2_s = obs_s_set(i) + obs_length/2;
    obs_p2_l = obs_l_set(i) - obs_width/2;
    obs_p3_s = obs_s_set(i) - obs_length/2;
    obs_p3_l = obs_l_set(i) + obs_width/2;
    obs_p4_s = obs_s_set(i) - obs_length/2;
    obs_p4_l = obs_l_set(i) - obs_width/2;
    obs_area_s = [obs_p1_s;obs_p2_s;obs_p4_s;obs_p3_s];
    obs_area_l = [obs_p1_l;obs_p2_l;obs_p4_l;obs_p3_l];
    fill(obs_area_s,obs_area_l,[0 0 0]);
end

== matlab function testEmplanner_cs -copy/Audi_A8_Sedan_1/decision&planning module/EM Planner/obs/MATLAB Function5 ==
  data: x_set input; match_point_index_set output; y_set input; frenet_path_x input; frenet_path_y input; frenet_path_heading input; frenet_path_kappa input; proj_x_set output; proj_y_set output; proj_heading_set output; proj_kappa_set output
function [match_point_index_set,proj_x_set,proj_y_set,proj_heading_set,proj_kappa_set] = ...
	fcn(x_set,y_set,frenet_path_x,frenet_path_y,frenet_path_heading,frenet_path_kappa)
	
%该函数将批量计算x_set,y_set中(x,y) 在frenet坐标系下的投影信息
%输入： x_set，y_set 待投影的点的集合
	%x_set,y_set,frenet_path_x,frenet_path_y,frenet_path_heading,frenet_path_kappa
	%曲线在直角坐标系下的x,y,heading,kappa
%输出：math_point_index_set 匹配点在frenet_path下的编号的集合（即从全局路径的第一个点开始数，第几个点是匹配点）

%由于事先不知道x_set中有多少个点需要投影，因此事先声明一个最大数量的点作为缓冲

n = 128;
%并且不知道投影点的数量，所以也不知道输出的数量，因此输出也要做缓冲，用nan表示不存在的点
%初始化输出最多为128个点。
%输出初始化
match_point_index_set = ones(n,1) * nan;
proj_x_set = ones(n,1) * nan;
proj_y_set = ones(n,1) * nan;
proj_heading_set = ones(n,1) * nan;
proj_kappa_set = ones(n,1) * nan;

%找匹配点，需要利用上一个周期的结果作为下一个周期遍历的起点，因此需要声明两个全局变量
persistent is_first_run;
persistent pre_match_point_index_set;
persistent pre_frenet_path_x;
persistent pre_frenet_path_y;
persistent pre_frenet_path_heading;
persistent pre_frenet_path_kappa;

%算法主函数入口

if isempty(is_first_run)
	% 该if分支表示函数首次运行
	is_first_run = 0; %赋值
	pre_frenet_path_x = frenet_path_x;
	pre_frenet_path_y = frenet_path_y;
	pre_frenet_path_heading = frenet_path_heading;
	pre_frenet_path_kappa = frenet_path_kappa;
	%记录首次运行计算的匹配点的结果供下个周期运行，先初始化
	pre_match_point_index_set = ones(n,1) * nan;
	
	%对x_set,y_set的点做遍历，找到他们的匹配点
	for i = 1 : length(x_set)
        if isnan(x_set(i))
            break;
        end
		%首次运行时，没有任何提示，只能从frenet_path的第一个点开始找
		start_search_index = 1;
		%声明increa_count,用于表示在遍历时distance连续增大的次数
		increase_count = 0;
		%开始遍历
		min_distance = inf;
		for j = start_search_index : length(frenet_path_x)
			distance = (x_set(i) - frenet_path_x(j))^2 + (y_set(i) - frenet_path_y(j))^2;
			%处理最小值
			if distance < min_distance
				min_distance = distance;
				match_point_index_set(i) = j; %math_point_index_set存放匹配点的序号
				increase_count = 0;
			else
				increase_count = increase_count + 1;
			end
			% 如果连续distanc增加50次,就不要再遍历了，节省时间
			if increase_count > 50 
				break;
			end	
		end
		%如何通过匹配点计算投影点，参考《自动驾驾驶控制算法第七讲》
		%或者《自动驾驶决策规划算法》第一章第三节
		
		%取出匹配点的编号
		match_point_index = match_point_index_set(i);
		
		%取出匹配点信息
		match_point_x = frenet_path_x(match_point_index);
		match_point_y = frenet_path_y(match_point_index);
		match_point_heading = frenet_path_heading(match_point_index);
		match_point_kappa = frenet_path_kappa(match_point_index);
		
		% 计算匹配点的位置向量和方向向量
		vector_match_point = [match_point_x;match_point_y];%位置向量
		vector_match_point_direction = [cos(match_point_heading);sin(match_point_heading)];%方向向量，全局坐标系下（大地坐标系）
		
		%声明待投影点的位矢
		vector_r = [x_set(i);y_set(i)];
		
		%通过匹配点计算投影点
		vector_d = vector_r - vector_match_point;
		ds = vector_d' * vector_match_point_direction;
		vector_proj_point = vector_match_point + vector_match_point_direction *ds;
		proj_heading = match_point_heading + match_point_kappa * ds;
		proj_kappa = match_point_kappa;
		
		%计算结果输出 
		proj_x_set(i) = vector_proj_point(1);
		proj_y_set(i) = vector_proj_point(2);
		proj_heading_set(i) = proj_heading;
		proj_kappa_set(i) = proj_kappa;
	end
	
	%匹配点的计算结果保存，供下一个周期使用
	pre_match_point_index_set = match_point_index_set;
else
	% 此分支不是首次运行
	
	%对每个x_set上的点做处理
	for i = 1 : length(x_set)
		%不是首次运行，对于点x_set(i),y_set(i)来说，start_search_index = pre_match_point_index_set(i)
		start_search_index = pre_match_point_index_set(i);%上个周期匹配点的编号作为本周期搜索的起点
		
        %
        % 对于障碍物的检测而言，当感知第一次检测到障碍物时，算法并不是首次运行，此时
        % pre_match_point_set的值是nan，如果还用上一个时刻的结果作为本周期搜索的起点
        % 必然会出问题，所以要修改
        % 声明 increase_count_limit
        increase_count_limit = 5;
        if isnan(start_search_index)
	        % 没有上个周期的结果，那么就不能只检查5次
	        increase_count_limit = 50;
	        % 搜索的起点也要设为 1
	        start_search_index = 1;
        end
		%声明increa_count,用于表示在遍历时distance连续增大的次数
		increase_count = 0;
		%开始遍历
		
		%这里多了一个步骤，判断遍历的方向
		%计算上个周期匹配点的位失
		vector_pre_match_point = [pre_frenet_path_x(start_search_index); pre_frenet_path_y(start_search_index)];
		vector_pre_match_point_direction = ...
			[cos(pre_frenet_path_heading(start_search_index));sin(pre_frenet_path_heading(start_search_index))];
		
		% 判断遍历的方向
		flag = ([x_set(i);y_set(i)] - vector_pre_match_point)' * vector_pre_match_point_direction;
		
		min_distance = inf;
		
		if flag > 0.001 
			for j = start_search_index : length(frenet_path_x)
				distance = (x_set(i) - frenet_path_x(j))^2 + (y_set(i) - frenet_path_y(j))^2;
				%处理最小值
				if distance < min_distance
					min_distance = distance;
					match_point_index_set(i) = j; %math_point_index_set存放匹配点的序号
					increase_count = 0;
				else
					increase_count = increase_count + 1;
				end
				% 如果连续distanc增加increase_count_limit次,就不要再遍历了，节省时间
				if increase_count > increase_count_limit
					break;
				end
			end
		elseif flag < -0.001
			for j = start_search_index :-1: 1
				distance = (x_set(i) - frenet_path_x(j))^2 + (y_set(i) - frenet_path_y(j))^2;
				%处理最小值
				if distance < min_distance
					min_distance = distance;
					match_point_index_set(i) = j; %math_point_index_set存放匹配点的序号
					increase_count = 0;
				else
					increase_count = increase_count + 1;
				end
				% 如果连续distanc增加50次,就不要再遍历了，节省时间
				if increase_count > increase_count_limit 
					break;
				end
			end
		else
			match_point_index_set(i) = start_search_index;
		end
			
		%如何通过匹配点计算投影点，参考《自动驾驾驶控制算法第七讲》
		%或者《自动驾驶决策规划算法》第一章第三节
		
		%取出匹配点的编号
		match_point_index = match_point_index_set(i);
		
		%取出匹配点信息
		match_point_x = frenet_path_x(match_point_index);
		match_point_y = frenet_path_y(match_point_index);
		match_point_heading = frenet_path_heading(match_point_index);
		match_point_kappa = frenet_path_kappa(match_point_index);
		
		% 计算匹配点的位置向量和方向向量
		vector_match_point = [match_point_x;match_point_y];%位置向量
		vector_match_point_direction = [cos(match_point_heading);sin(match_point_heading)];%方向向量
		
		%声明待投影点的位矢
		vector_r = [x_set(i);y_set(i)];
		
		%通过匹配点计算投影点
		vector_d = vector_r - vector_match_point;
		ds = vector_d' * vector_match_point_direction;
		vector_proj_point = vector_match_point + ds * vector_match_point_direction;
		proj_heading = match_point_heading + match_point_kappa * ds;
		proj_kappa = match_point_kappa;
		
		%计算结果输出 
		proj_x_set(i) = vector_proj_point(1);
		proj_y_set(i) = vector_proj_point(2);
		proj_heading_set(i) = proj_heading;
		proj_kappa_set(i) = proj_kappa;
	end
	
	%匹配点的计算结果保存，供下一个周期使用
	pre_match_point_index_set = match_point_index_set;
	pre_frenet_path_x = frenet_path_x;
	pre_frenet_path_y = frenet_path_y;
	pre_frenet_path_heading = frenet_path_heading;
	pre_frenet_path_kappa = frenet_path_kappa;
end

== matlab function testEmplanner_cs -copy/Audi_A8_Sedan_1/decision&planning module/EM Planner/calc speed planning start condition ==
  data: plan_start_vx input; plan_start_s_dot output; plan_start_vy input; plan_start_ax input; plan_start_ay input; plan_start_heading input; plan_start_s_dot2 output
function [plan_start_s_dot,plan_start_s_dot2] = fcn(plan_start_vx,plan_start_vy,plan_start_ax,plan_start_ay,plan_start_heading)
% 该函数计算速度规划的初始条件
tor = [cos(plan_start_heading);sin(plan_start_heading)];
v_t = tor'*[plan_start_vx;plan_start_vy];
a_t = tor'*[plan_start_ax;plan_start_ay];
plan_start_s_dot = v_t;
plan_start_s_dot2 = a_t;

== matlab function testEmplanner_cs -copy/Audi_A8_Sedan_1/decision&planning module/EM Planner/simple speed qp planning ==
  data: plan_start_s_dot input; s_init output; plan_start_s_dot2 input; s_end input; recommend_T input; s_dot_init output; s_dot2_init output; relative_time_init output
function [s_init,s_dot_init,s_dot2_init,relative_time_init] = fcn(plan_start_s_dot,plan_start_s_dot2,s_end,recommend_T)
%简单速度二次规划
coder.extrinsic("quadprog")
n = 51;
s_init = zeros(n,1);
s_dot_init = zeros(n,1);
s_dot2_init = zeros(n,1);
relative_time_init = zeros(n,1);

Aeq = zeros(3*n,2*n - 2);
beq = zeros(2*n - 2,1);
lb = ones(3*n,1);
ub = lb;
dt = recommend_T/(n-1);
A_sub =[1,0;
        dt,1;
        (1/3)*dt^2,(1/2)*dt;
        -1,0;
        0,-1;
        (1/6)*dt^2,dt/2];
for i = 1:n - 1
    Aeq(3*i-2:3*i+3,2*i-1:2*i) = A_sub;
end

for i = 1:n
   lb(3*i - 2) = -inf;
   lb(3*i - 1) = 0;
   lb(3*i) = -8;
   ub(3*i - 2) = inf;
   ub(3*i - 1) = 50;
   ub(3*i) = 2;
end
lb(1) = 0;
lb(2) = plan_start_s_dot;
lb(3) = plan_start_s_dot2;
ub(1) = lb(1);
ub(2) = lb(2);
ub(3) = lb(3);
lb(3*n - 2) = s_end;
ub(3*n - 2) = s_end;
A3 = zeros(3*n,3*n);
A4 = zeros(3*n,n - 1);
A4_sub =[0;0;1;0;0;-1];
for i = 1:n - 1
   A3(3*i,3*i) = 1;
   A4(3*i-2:3*i+3,i:i) = A4_sub;
end
A3(3*n,3*n) = 1;
H = A3 + 100*(A4*A4');
H = 2*H;
f = zeros(3*n,1);
X = quadprog(H,f,[],[],Aeq',beq,lb,ub);
for i = 1:n
   s_init(i) = X(3*i - 2);
   s_dot_init(i) = X(3*i - 1);
   s_dot2_init(i) = X(3*i);
   relative_time_init(i) = (i - 1)*dt;
end

== matlab function testEmplanner_cs -copy/Audi_A8_Sedan_1/decision&planning module/referenceline provider/MATLAB Function2 ==
  data: host_match_point_index input; referenceline_x_init output; global_path_x input; global_path_y input; referenceline_y_init output
function [referenceline_x_init,referenceline_y_init] = fcn(host_match_point_index,global_path_x,global_path_y)

%该函数将在全局路径上提取referenceline的未平滑的初值
%输入：host_match_point_index 自车的位置在全局路径的匹配点的编号
% global_path_x,global_path_y 全局路径数据

%输出：referenceline_x_init,referenceline_y_init 未平滑的参考线的xy坐标

%由于global_path是每1m取一个点，所以从匹配点I往后取30个点，往前取150个点，一共181个点
%如果前面不够的话，就用后面补，后面不够的话就从前面补，保证总数为181个点。

%索引初始化

start_index = -1;

%判断后面前面的点是否足够多
if host_match_point_index - 30 < 1
	%匹配点前面的数太少了，发生在刚开始
	start_index = 1;
elseif host_match_point_index + 150 > length(global_path_x)
	%匹配点后面的点太少了，发生在结束位置
	start_index = length(global_path_x) - 180;
else 
	%匹配点正常
	start_index = host_match_point_index - 30;
end

%提取reference_line
referenceline_x_init = global_path_x(start_index:start_index+180);%提取，类似于切片
referenceline_y_init = global_path_y(start_index:start_index+180);

== matlab function testEmplanner_cs -copy/Audi_A8_Sedan_2/PathFollower_Preview_1/LateralController/CTRL REFERENCES/Calculate Lateral Error/eml_find_10k_lateral_error_points ==
  data: pvp input size=2; dist_psvehicle output size=10; TrajOffset_x_y_Y input size=3; ActorOffset_Left_Right input; p0 input size=2; PreviewDistance input size=10; Traj_x parameter; Traj_y parameter; Traj_t parameter; Traj_v parameter; RefreshCounter parameter
function dist_psvehicle  = eml_find_10k_lateral_error_points(pvp,TrajOffset_x_y_Y,ActorOffset_Left_Right,p0,PreviewDistance,Traj_x,Traj_y,Traj_t,Traj_v,RefreshCounter)

dist_psvehicle = emlfcn_find_10k_lateral_error_points(pvp,TrajOffset_x_y_Y,ActorOffset_Left_Right,p0,PreviewDistance,Traj_x,Traj_y,Traj_t,Traj_v,RefreshCounter);

% end function

== matlab function testEmplanner_cs -copy/Audi_A8_Sedan_1/control module/control main/longitudinal control double PID/MATLAB Function1 ==
  data: u input; throttle output; brake output
function [throttle,brake] = fcn(u)
    if u>=0
        throttle=u;
        brake=0;
    else
        throttle=0;
        brake=-u;
    end
